simulink model "ftc_4AGENTS_sim_test"  (R2024a)
settings: Solver=VariableStepAuto  StartTime=0.0  StopTime=10  FixedStep=0.001  RelTol=1e-3
undefined symbols (not defined in the file or in its folder): param, pos_init
libraries: sim3dlib x5
settings Model: PacingRate=0.100000  Creator=antor  LastModifiedBy=antor

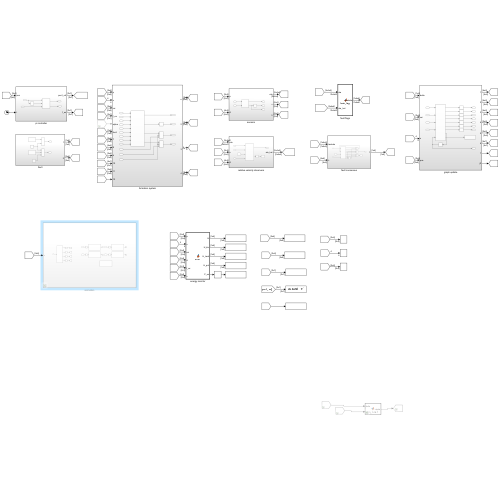
[thumbnail: Simulink's stored preview of the top-level diagram]
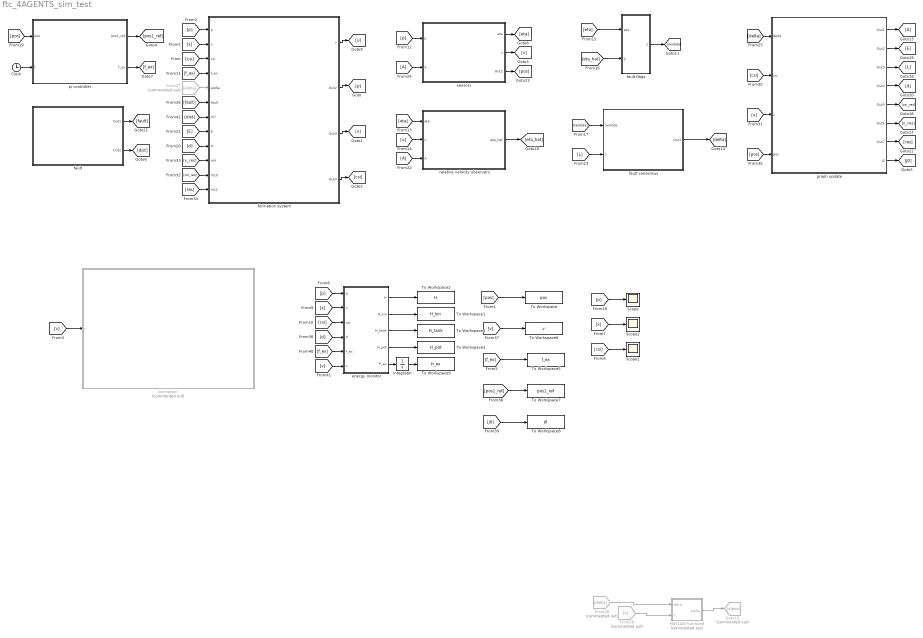
== system ftc_4AGENTS_sim_test ==
  Clock : Clock
  From22 : From
  From24 : From
  From27 : From  Commented=on  GotoTag=alpha
  From28 : From  Commented=on  GotoTag=delta
  From29 : From  Commented=on  GotoTag=x
  Goto13 : Goto
  Goto15 : Goto  Commented=on  GotoTag=alpha
  Integrator : Integrator
  MATLAB Function8 : MATLAB Function  Commented=on  TreatAsAtomicUnit=on
  Scope : Scope
  Scope1 : Scope
  Scope2 : Scope
  To Workspace : ToWorkspace  VariableName=pos  SaveFormat=Timeseries  SampleTime=param.T
  To Workspace1 : ToWorkspace  VariableName=H_kin  SaveFormat=Timeseries  SampleTime=param.T
  To Workspace2 : ToWorkspace  VariableName=H  SaveFormat=Timeseries  SampleTime=param.T
  To Workspace3 : ToWorkspace  VariableName=H_pot  SaveFormat=Timeseries  SampleTime=param.T
  To Workspace4 : ToWorkspace  VariableName=H_tank  SaveFormat=Timeseries  SampleTime=param.T
  To Workspace5 : ToWorkspace  VariableName=f_ex  SaveFormat=Timeseries  SampleTime=param.T
  To Workspace6 : ToWorkspace  VariableName=v  SaveFormat=Timeseries  SampleTime=param.T
  To Workspace7 : ToWorkspace  VariableName=pos1_ref  SaveFormat=Timeseries  SampleTime=param.T
  To Workspace8 : ToWorkspace  VariableName=j0  SaveFormat=Timeseries  SampleTime=param.T
  To Workspace9 : ToWorkspace  VariableName=H_ex  SaveFormat=Timeseries  SampleTime=param.T
  animation : Subsystem  Commented=on
  energy monitor : MATLAB Function  TreatAsAtomicUnit=on
  fault : Subsystem
  fault consensus : Subsystem
  fault flags : MATLAB Function  TreatAsAtomicUnit=on
  formation system : Subsystem
  graph update : Subsystem
  pi controller : Subsystem
  relative velocity observers : Subsystem
  sensors : Subsystem
  wires:
  energy monitor/1(H) -> To Workspace2/1
  energy monitor/2(H_kin) -> To Workspace1/1
  energy monitor/4(H_pot) -> To Workspace3/1
  energy monitor/3(H_tank) -> To Workspace4/1
  [x] -> energy monitor/2(x)
  [csi] -> energy monitor/3(csi)
  [p] -> energy monitor/1(p)
  [eta] -> fault flags/1(eta)
  [eta_hat] -> fault flags/2(eta_hat)
  fault flags/1(lambda) -> [lambda]
  MATLAB Function8/1(alpha) -> Goto15/1
  From28/1 -> MATLAB Function8/1(delta)
  From29/1 -> MATLAB Function8/2(x)
  [d] -> energy monitor/4(d)
  [lambda] -> fault consensus/1(lambda)
  [L] -> fault consensus/2(L)
  fault consensus/1(Out1) -> [delta]
  [eta] -> relative velocity observers/1(eta)
  [u] -> relative velocity observers/2(u)
  From22/1 -> relative velocity observers/3(A)
  relative velocity observers/1(eta_hat) -> [eta_hat]
  [p] -> sensors/1(p)
  From24/1 -> sensors/2(A)
  sensors/1(eta) -> [eta]
  sensors/3(Out2) -> [pos]
  [pos] -> pi controller/1(pos)
  Clock/1 -> pi controller/2(t)
  pi controller/2(f_ex) -> [f_ex]
  [p] -> formation system/1(p)
  [x] -> formation system/2(x)
  [csi] -> formation system/3(csi)
  [f_ex] -> formation system/4(f_ex)
  From27/1 -> formation system/5(alpha)
  [fault] -> formation system/6(fault)
  [E] -> formation system/8(E)
  [d] -> formation system/9(d)
  [x_res] -> formation system/10(In9)
  [csi_res] -> formation system/11(In10)
  [res] -> formation system/12(In11)
  formation system/1(u) -> [u]
  formation system/2(Out2) -> [p]
  formation system/3(Out3) -> [x]
  formation system/4(Out4) -> [csi]
  [delta] -> graph update/1(delta)
  [csi] -> graph update/2(csi)
  [x] -> graph update/3(x)
  [pos] -> graph update/4(pos)
  graph update/1(Out1) -> Goto13/1
  graph update/2(Out2) -> [E]
  graph update/3(Out3) -> [L]
  graph update/4(Out4) -> [d]
  graph update/5(Out5) -> [csi_res]
  graph update/6(Out6) -> [x_res]
  graph update/7(Out7) -> [res]
  [v] -> animation/1(v)
  [pos] -> To Workspace/1
  [f_ex] -> To Workspace5/1
  [p] -> Scope/1
  [x] -> Scope2/1
  [csi] -> Scope1/1
  sensors/2(v) -> [v]
  [v] -> To Workspace6/1
  pi controller/1(pos1_ref) -> [pos1_ref]
  [pos1_ref] -> To Workspace7/1
  graph update/8(j0) -> [j0]
  [j0] -> To Workspace8/1
  [v] -> energy monitor/6(v)
  [f_ex] -> energy monitor/5(f_ex)
  energy monitor/5(P_ex) -> Integrator/1
  Integrator/1 -> To Workspace9/1
  fault/1(Out1) -> [fault]
  fault/2(Out2) -> [dist]
  [dist] -> formation system/7(In7)

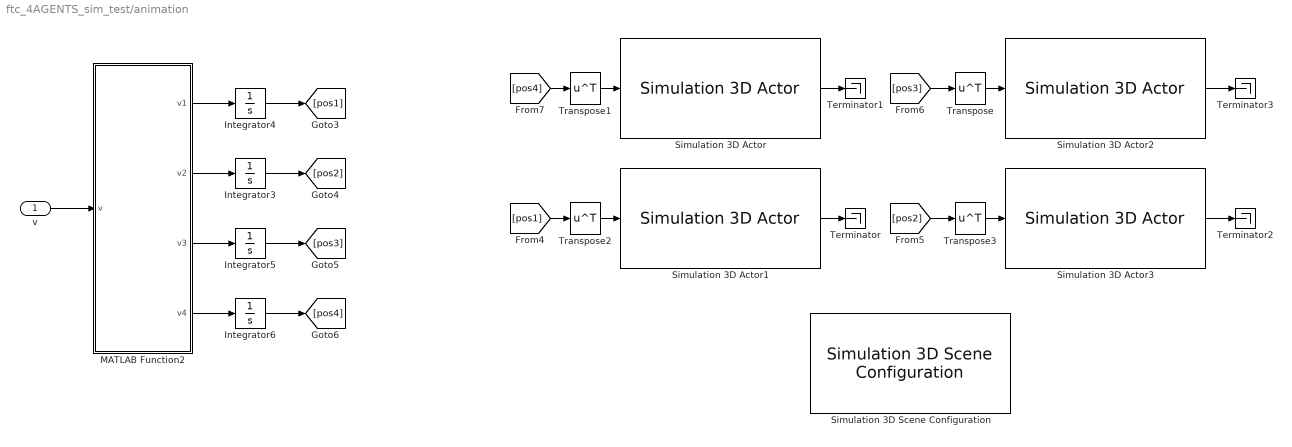
== system ftc_4AGENTS_sim_test/animation ==
  v : Inport
  Integrator3 : Integrator  InitialCondition=[pos_init(:, 2); 0]
  Integrator4 : Integrator  InitialCondition=[pos_init(:, 1); 0]
  Integrator5 : Integrator  InitialCondition=[pos_init(:, 3); 0]
  Integrator6 : Integrator  InitialCondition=[pos_init(:, 4); 0]
  MATLAB Function2 : MATLAB Function  TreatAsAtomicUnit=on
  Simulation 3D Actor : sim3dlib/Simulation 3D Actor  Priority=1  ActorName=actor4  ParentName=Scene Origin  Operation=Create at setup  InitScriptText=|  SampleTime=-1  Translation=single([0 0 0])  Rotation=single([0 0 0])  Scale=single([1 1 1])  InputsText=actor4.Translation  aMode=5  ActorTag=actor4  ActorType=Sim3dActor  ID=C
      | Actor.createShape('sphere', [1 1 1]);
      | Actor.Scale = 0.1;
      | Actor.Color = [0 0 0];
  Simulation 3D Actor1 : sim3dlib/Simulation 3D Actor  Priority=1  ActorName=actor1  ParentName=Scene Origin  Operation=Create at setup  InitScriptText=|  SampleTime=-1  Translation=single([0 0 0])  Rotation=single([0 0 0])  Scale=single([1 1 1])  InputsText=actor1.Translation  aMode=5  ActorTag=actor1  ActorType=Sim3dActor  ID=C
      | Actor.createShape('sphere', [1 1 1]);
      | Actor.Scale = 0.1;
      | Actor.Color = [0 0 1];
  Simulation 3D Actor2 : sim3dlib/Simulation 3D Actor  Priority=1  ActorName=actor3  ParentName=Scene Origin  Operation=Create at setup  InitScriptText=|  SampleTime=-1  Translation=single([0 0 0])  Rotation=single([0 0 0])  Scale=single([1 1 1])  InputsText=actor3.Translation  aMode=5  ActorTag=actor3  ActorType=Sim3dActor  ID=C
      | Actor.createShape('sphere', [1 1 1]);
      | Actor.Scale = 0.1;
      | Actor.Color = [0 0 0];
  Simulation 3D Actor3 : sim3dlib/Simulation 3D Actor  Priority=1  ActorName=actor2  ParentName=Scene Origin  Operation=Create at setup  InitScriptText=|  SampleTime=-1  Translation=single([0 0 0])  Rotation=single([0 0 0])  Scale=single([1 1 1])  InputsText=actor2.Translation  aMode=5  ActorTag=actor2  ActorType=Sim3dActor  ID=C
      | Actor.createShape('sphere', [1 1 1]);
      | Actor.Scale = 0.1;
      | Actor.Color = [0 0 0];
  Simulation 3D Scene Configuration : sim3dlib/Simulation 3D Scene Configuration  Priority=0  ProjectFormat=Default Scenes  SceneDesc=Empty scene  ProjectName=C:\Program Files\MATLAB\R2024a\toolbox\shared\sim3d_projects\automotive_project_windows\UE\WindowsNoEditor\VehicleSimulation.exe  ScenePath=/Game/Maps/HwStrght  EnableOpenDRIVE=off  vehTagList={'Custom';'Scene Origin';'actor1';'actor2';'actor3';'actor4'}  vehTag=Scene Origin  FreeCameraInitialTranslation=[2.5, 2.5, 15]  FreeCameraDefaultInitialTranslation=[-6, 0, 2]  FreeCameraInitialRotation=[90, -90, 0]  FreeCameraDefaultInitialRotation=[0, -15, 0]  OpVisEn=off  Ts=.02  EnableWindow=on  EnableRemoteAccess=off  EnableWeather=off  SunAzimuth=90  SunAltitude=40.0  EnableGeospatialSun=off  Latitude=0  Longitude=0  Date=2023-01-01  Time=10:30:00  GeoTimeZone=-5.0  SunDaylightSaving=off  wind=1  clouds=10  EnableVolumetricClouds=off  CloudCoverage=0  CloudAltitude=6  fog=0  rain=0  RaindropsEffect=off  SnowDensity=0  EnableGeospatial=off  UseTrueOrigin=off  OriginHeight=200  OriginLatitude=40.744652  OriginLongitude=-73.988864  MapStyle=Aerial  AdditionalAssetIDs=[]  UseAdvancedSunSky=off  SolarTime=11  TimeZone=-5  Day=21  Month=9  Year=2022  UseDaylightSavingTime=on  DSTStartDay=10  DSTStartMonth=3  DSTEndDay=3  DSTEndMonth=11  DSTSwitchHour=2  sensorTag=MainCamera1  sensorId=1  sensorName=MainCamera1  mountLoc=Origin  offsetFlag=off  tmountOffset=[0, 0, 0]  rmountOffset=[0, 0, 0]  HorizontalResolution=1280  VerticalResolution=720  HorizontalFOV=60  mountPoint=[0 0 0]  mountOrientation=[0 0 0]  aMode=5  ID=1  GeoTrigger=Inactive
      settings: LibrarySourceBlock=sl3dlib/Simulation 3D/Environment/Simulation 3D Scene Configuration
  Terminator{,1..3} (4 alike) : Terminator
  Transpose{,1..3} (4 alike) : Math  Operator=transpose
  wires:
  MATLAB Function2/2(v2) -> Integrator3/1
  Simulation 3D Actor/1 -> Terminator1/1
  [pos2] -> Transpose3/1
  Integrator5/1 -> [pos3]
  Integrator6/1 -> [pos4]
  [pos1] -> Transpose2/1
  Integrator4/1 -> [pos1]
  Integrator3/1 -> [pos2]
  MATLAB Function2/1(v1) -> Integrator4/1
  Simulation 3D Actor3/1 -> Terminator2/1
  MATLAB Function2/3(v3) -> Integrator5/1
  Transpose3/1 -> Simulation 3D Actor3/1
  Transpose2/1 -> Simulation 3D Actor1/1
  Transpose/1 -> Simulation 3D Actor2/1
  Transpose1/1 -> Simulation 3D Actor/1
  MATLAB Function2/4(v4) -> Integrator6/1
  Simulation 3D Actor2/1 -> Terminator3/1
  [pos4] -> Transpose1/1
  [pos3] -> Transpose/1
  Simulation 3D Actor1/1 -> Terminator/1
  v/1 -> MATLAB Function2/1(v)

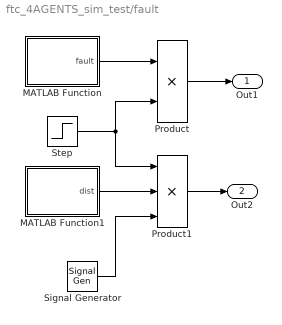
== system ftc_4AGENTS_sim_test/fault ==
  MATLAB Function : MATLAB Function  TreatAsAtomicUnit=on
  MATLAB Function1 : MATLAB Function  TreatAsAtomicUnit=on
  Product : Product
  Product1 : Product  Inputs=3
  Signal Generator : SignalGenerator  WaveForm=random  Frequency=0.2  Units=rad/sec
  Step : Step  Time=param.fault_time+100  SampleTime=0
  Out1 : Outport
  Out2 : Outport  Port=2
  wires:
  Step/1 -> Product1/1, Product/2
  MATLAB Function/1(fault) -> Product/1
  Product/1 -> Out1/1
  MATLAB Function1/1(dist) -> Product1/2
  Product1/1 -> Out2/1
  Signal Generator/1 -> Product1/3

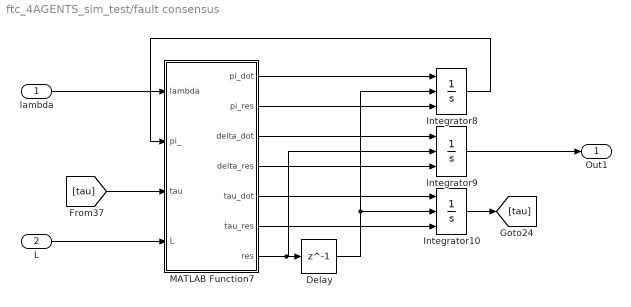
== system ftc_4AGENTS_sim_test/fault consensus ==
  lambda : Inport
  L : Inport  Port=2
  Delay : Delay  DelayLength=1
  Integrator10 : Integrator  ExternalReset=rising  InitialConditionSource=external
  Integrator8 : Integrator  ExternalReset=rising  InitialConditionSource=external
  Integrator9 : Integrator  ExternalReset=rising  InitialConditionSource=external
  MATLAB Function7 : MATLAB Function  TreatAsAtomicUnit=on
  Out1 : Outport
  wires:
  MATLAB Function7/3(delta_dot) -> Integrator9/1
  MATLAB Function7/7(res) -> Integrator9/2, Delay/1
  MATLAB Function7/1(pi_dot) -> Integrator8/1
  MATLAB Function7/6(tau_res) -> Integrator10/3
  MATLAB Function7/5(tau_dot) -> Integrator10/1
  Integrator9/1 -> Out1/1
  MATLAB Function7/2(pi_res) -> Integrator8/3
  Integrator8/1 -> MATLAB Function7/2(pi_)
  Delay/1 -> Integrator8/2, Integrator10/2
  MATLAB Function7/4(delta_res) -> Integrator9/3
  Integrator10/1 -> [tau]
  [tau] -> MATLAB Function7/3(tau)
  L/1 -> MATLAB Function7/4(L)
  lambda/1 -> MATLAB Function7/1(lambda)

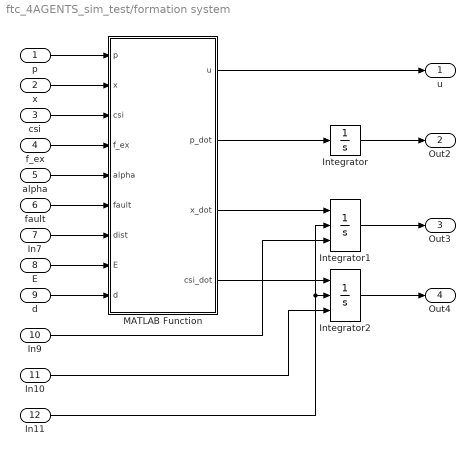
== system ftc_4AGENTS_sim_test/formation system ==
  p : Inport
  x : Inport  Port=2
  csi : Inport  Port=3
  f_ex : Inport  Port=4
  alpha : Inport  Port=5
  fault : Inport  Port=6
  In7 : Inport  Port=7
  E : Inport  Port=8
  d : Inport  Port=9
  In9 : Inport  Port=10
  In10 : Inport  Port=11
  In11 : Inport  Port=12
  Integrator : Integrator  InitialCondition=zeros(2, param.N)
  Integrator1 : Integrator  ExternalReset=rising  InitialConditionSource=external  InitialCondition=50*ones(1, param.N)
  Integrator2 : Integrator  ExternalReset=rising  InitialConditionSource=external  InitialCondition=param.csi_init
  MATLAB Function : MATLAB Function  TreatAsAtomicUnit=on
  u : Outport
  Out2 : Outport  Port=2
  Out3 : Outport  Port=3
  Out4 : Outport  Port=4
  wires:
  MATLAB Function/2(p_dot) -> Integrator/1
  MATLAB Function/4(csi_dot) -> Integrator2/1
  MATLAB Function/3(x_dot) -> Integrator1/1
  f_ex/1 -> MATLAB Function/4(f_ex)
  E/1 -> MATLAB Function/8(E)
  In11/1 -> Integrator1/2, Integrator2/2
  In9/1 -> Integrator1/3
  Integrator/1 -> Out2/1
  alpha/1 -> MATLAB Function/5(alpha)
  d/1 -> MATLAB Function/9(d)
  fault/1 -> MATLAB Function/6(fault)
  Integrator2/1 -> Out4/1
  x/1 -> MATLAB Function/2(x)
  MATLAB Function/1(u) -> u/1
  p/1 -> MATLAB Function/1(p)
  In10/1 -> Integrator2/3
  csi/1 -> MATLAB Function/3(csi)
  Integrator1/1 -> Out3/1
  In7/1 -> MATLAB Function/7(dist)

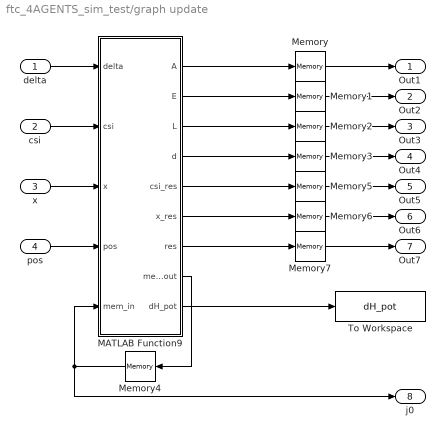
== system ftc_4AGENTS_sim_test/graph update ==
  delta : Inport
  csi : Inport  Port=2
  x : Inport  Port=3
  pos : Inport  Port=4
  MATLAB Function9 : MATLAB Function  TreatAsAtomicUnit=on
  Memory : Memory  InitialCondition=param.A
  Memory1 : Memory  InitialCondition=param.E
  Memory2 : Memory  InitialCondition=param.L
  Memory3 : Memory  InitialCondition=param.d
  Memory4 : Memory
  Memory5 : Memory  InitialCondition=param.csi_init
  Memory6 : Memory  InitialCondition=param.x_init
  Memory7 : Memory
  To Workspace : ToWorkspace  VariableName=dH_pot  SaveFormat=Timeseries  SampleTime=-1
  Out1 : Outport
  Out2 : Outport  Port=2
  Out3 : Outport  Port=3
  Out4 : Outport  Port=4
  Out5 : Outport  Port=5
  Out6 : Outport  Port=6
  Out7 : Outport  Port=7
  j0 : Outport  Port=8
  wires:
  MATLAB Function9/1(A) -> Memory/1
  Memory/1 -> Out1/1
  MATLAB Function9/3(L) -> Memory2/1
  Memory4/1 -> j0/1, MATLAB Function9/5(mem_in)
  MATLAB Function9/5(csi_res) -> Memory5/1
  MATLAB Function9/6(x_res) -> Memory6/1
  MATLAB Function9/2(E) -> Memory1/1
  MATLAB Function9/4(d) -> Memory3/1
  MATLAB Function9/8(mem_out) -> Memory4/1
  Memory1/1 -> Out2/1
  Memory3/1 -> Out4/1
  MATLAB Function9/7(res) -> Memory7/1
  Memory2/1 -> Out3/1
  x/1 -> MATLAB Function9/3(x)
  Memory6/1 -> Out6/1
  Memory5/1 -> Out5/1
  csi/1 -> MATLAB Function9/2(csi)
  Memory7/1 -> Out7/1
  delta/1 -> MATLAB Function9/1(delta)
  pos/1 -> MATLAB Function9/4(pos)
  MATLAB Function9/9(dH_pot) -> To Workspace/1

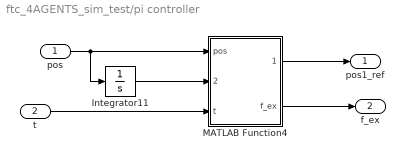
== system ftc_4AGENTS_sim_test/pi controller ==
  pos : Inport
  t : Inport  Port=2
  Integrator11 : Integrator
  MATLAB Function4 : MATLAB Function  TreatAsAtomicUnit=on
  pos1_ref : Outport
  f_ex : Outport  Port=2
  wires:
  t/1 -> MATLAB Function4/3(t)
  pos/1 -> Integrator11/1, MATLAB Function4/1(pos)
  Integrator11/1 -> MATLAB Function4/2(pos_int)
  MATLAB Function4/2(f_ex) -> f_ex/1
  MATLAB Function4/1(pos1_ref) -> pos1_ref/1

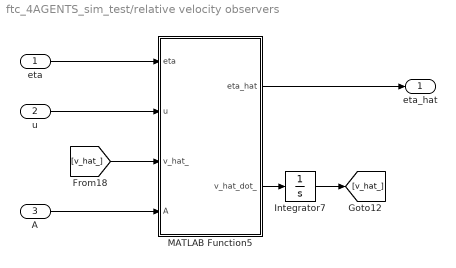
== system ftc_4AGENTS_sim_test/relative velocity observers ==
  eta : Inport
  u : Inport  Port=2
  A : Inport  Port=3
  Integrator7 : Integrator  InitialCondition=zeros(2*param.N, param.N)
  MATLAB Function5 : MATLAB Function  TreatAsAtomicUnit=on
  eta_hat : Outport
  wires:
  MATLAB Function5/1(eta_hat) -> eta_hat/1
  [v_hat_] -> MATLAB Function5/3(v_hat_)
  A/1 -> MATLAB Function5/4(A)
  eta/1 -> MATLAB Function5/1(eta)
  u/1 -> MATLAB Function5/2(u)
  Integrator7/1 -> [v_hat_]
  MATLAB Function5/2(v_hat_dot_) -> Integrator7/1

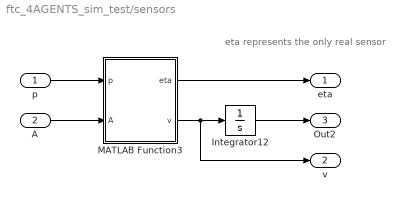
== system ftc_4AGENTS_sim_test/sensors ==
  note: eta represents the only real sensor
  p : Inport
  A : Inport  Port=2
  Integrator12 : Integrator  InitialCondition=param.pos_init
  MATLAB Function3 : MATLAB Function  TreatAsAtomicUnit=on
  eta : Outport
  v : Outport  Port=2
  Out2 : Outport  Port=3
  wires:
  MATLAB Function3/2(v) -> v/1, Integrator12/1
  MATLAB Function3/1(eta) -> eta/1
  Integrator12/1 -> Out2/1
  p/1 -> MATLAB Function3/1(p)
  A/1 -> MATLAB Function3/2(A)

== matlab function ftc_4AGENTS_sim_test/fault flags ==
  data: eta input; lambda output; eta_hat input; param parameter
function lambda = fault_flag(eta, eta_hat, param)
    N = 4;
    theta = param.theta;

    lambda = zeros(1, N, N);
    
    for i = 1:N
        for j = 1:N
            lambda(:, i, j) = norm(eta(:, i, j) - eta_hat(:, i, j)) > theta;
        end
    end

    test = lambda(:, 1, :);
end

== matlab function ftc_4AGENTS_sim_test/fault consensus/MATLAB Function7 ==
  data: lambda input; pi_ input; tau input; L input; pi_dot output; pi_res output; delta_dot output; delta_res output; tau_dot output; tau_res output; param parameter; res output
function [pi_dot, pi_res, delta_dot, delta_res, tau_dot, tau_res, res] = fault_cons(lambda, pi_, tau, L, param)
    N = 4;
    tau_star = param.tau_star;

    pi_dot = zeros(N*N, 1);
    pi_dot(:, 1) = -2*kron(L, eye(N))*pi_;
    delta_dot = zeros(1, N);
    tau_dot = 1;

    temp = squeeze(lambda).';
    pi_res = temp(:);
    delta_res = zeros(1, N);
    for i = 1:N
        [max_delta, delta_res(i)] = max(pi_(((i-1)*N + 1):i*N));
        if max_delta <= 0.1
            delta_res(i) = 0;
        end
    end
    tau_res = 0;

    res = tau >= tau_star;
end

== matlab function ftc_4AGENTS_sim_test/MATLAB Function8 ==
  data: alpha output; delta input; x input; param parameter
function alpha = en_transf(delta, x, param)
    N = 4;

    j0 = delta(1);

    alpha = zeros(N, N);
    csi_init = param.csi_init;
    if j0 > 0.9
    %     n1 = mod(j0+N-2, N)+1;
    %     n2 = mod(j0, N)+1;
    %     n3 = mod(j0+1, N)+1;
    % 
    %     for i = 1:N
    %         if x(i) >= 1
    %             alpha(i, 1:3) = 0.00001;
    %         end
    %     end
    end

    
end

== matlab function ftc_4AGENTS_sim_test/graph update/MATLAB Function9 ==
  data: delta input; csi input; x input; pos input; mem_in input; param parameter; A output; E output; L output; d output; csi_res output; x_res output; res output; mem_out output; dH_pot output
function [A, E, L, d, csi_res, x_res, res, mem_out, dH_pot] = graph_upd(delta, csi, x, pos, mem_in, param)
    N = 4;
    pos_init = param.pos_init;
    K = param.K;

    j0 = delta(1);
    if mem_in ~= 0
        j0 = mem_in;
    end

    A = zeros(N);
    A(:, :) = param.A;
    E = zeros(N);
    E(:, :) = param.E;
    L = zeros(N);
    L(:, :) = param.L;
    d = zeros(2, N);
    d(:, :) = param.d;
    csi_res = zeros(2, N);
    csi_res(:, :) = param.csi_init;
    x_res = zeros(N, 1);
    x_res(:) = param.x_init;
    res = 0;
    mem_out = 0;
    dH_pot = 0;

    if j0 > 0.9
        mem_out = j0;

        n1 = mod(j0+N-2, N)+1;
        n2 = mod(j0, N)+1;
        n3 = mod(j0+1, N)+1;

        A_new = A;
        A_new(j0, :) = zeros(1, N);
        A_new(:, j0) = zeros(N, 1);

        temp = zeros(1, N);
        temp(n2) = 1;
        A_new(n1, :) = A_new(n1, :) + temp;
        A_new(:, n1) = A_new(:, n1) + temp.';

        edges = [];
        for i = 1:N
            for j = i+1:N
                if A_new(i, j) ~= 0
                    edges = [edges; i, j];
                end
            end
        end
        E_new = zeros(N);
        for k = 1:size(edges, 1)
            E_new(edges(k, 1), k) = -1;
            E_new(edges(k, 2), k) = 1;
        end

        L_new = diag(sum(A_new, 2)) - A_new;

        pos_rest = pos_init;
        pos_rest(:, n1) = pos_init(:, n1) + (pos_init(:, j0) - pos_init(:, n1))*cos(pi/3) + (pos_init(:, n3) - pos_init(:, n1))*(1-sin(pi/3));
        d_new = zeros(2, N);
        for j = 1:N
            for i = 1:N
                d_new(:, j) = d_new(:, j) + E_new(i, j)*pos_rest(:, i);
            end
        end

        dH_pot = 0;
        for j = 1:N
            dH_pot = dH_pot - 1/2*(csi(:, j)-d(:, j)).'*K(:, :, j)*(csi(:, j)-d(:, j));
        end 
        csi_res = zeros(2, N);
        for j = 1:N
            for i = 1:N
                csi_res(:, j) = csi_res(:, j) + E_new(i, j)*pos(:, i);
            end
        end
        for j = 1:N
            dH_pot = dH_pot + 1/2*(csi_res(:, j)-d_new(:, j)).'*K(:, :, j)*(csi_res(:, j)-d_new(:, j));
        end 
        res = 1;

        H_tank = zeros(1, N);
        for i = 1:N
            H_tank(i) = 1/2*x(i)^2;
        end        
        % for i = 1:N
        %     x_res(i) = sqrt(1/2*(H_tank-dH_pot));
        % end

        x_res(j0) = x(j0);
        x_res(n1) = sqrt(H_tank(n1) + H_tank(n2) - dH_pot);
        x_res(n2) = sqrt(H_tank(n1) + H_tank(n2) - dH_pot);
        x_res(n3) = x(n3);

        E = E_new;
        A = A_new;
        L = L_new;
        d = d_new;
    end
end

== matlab function ftc_4AGENTS_sim_test/fault/MATLAB Function ==
  data: fault output; param parameter
function fault = fault(param)
N = 4;
fault_i = param.fault_i;
fault_perc = param.fault_perc;

fault = zeros(1, N);
fault(fault_i) = fault_perc/100;
end

== matlab function ftc_4AGENTS_sim_test/fault/MATLAB Function1 ==
  data: dist output; param parameter
function dist = dist(param)
N = 4;
fault_i = param.fault_i;
dist_amp = param.dist_amp;

dist = zeros(2, N);
dist(:, fault_i) = dist_amp*rand(2, 1);
end

== matlab function ftc_4AGENTS_sim_test/energy monitor ==
  data: p input; H output; x input; csi input; d input; f_ex input; v input; H_kin output; H_tank output; H_pot output; param parameter; P_ex output
function [H, H_kin, H_tank, H_pot, P_ex] = ener(p, x, csi, d, f_ex, v, param)
    N = 4;
    M = param.M;
    K = param.K;

    H_kin = zeros(1, N);
    H_tank = zeros(1, N);
    H_pot = zeros(1, N);

    for i = 1:N
        H_kin(i) = 1/2*p(:, i).'*(M(:, :, i)\p(:, i));
        H_tank(i) = 1/2*x(i)*x(i);
    end

    for j = 1:N
        H_pot(j) = 1/2*(csi(:, j)-d(:, j)).'*K(:, :, j)*(csi(:, j)-d(:, j));
    end

    H = sum([H_kin; H_pot; H_tank], 1);

    P_ex = f_ex.'*v(:, 1);
end

== matlab function ftc_4AGENTS_sim_test/formation system/MATLAB Function ==
  data: p input; u output; p_dot output; x input; csi input; f_ex input; alpha input; fault input; dist input; E input; d input; x_dot output; csi_dot output; param parameter
function [u, p_dot, x_dot, csi_dot] = sys(p, x, csi, f_ex, alpha, fault, dist, E, d, param)
    N = 4;
    K = param.K;
    M = param.M;
    B = param.B;

    r = zeros(1, 2, N);
    h = zeros(1, 2, N, N);

    for i = 1:N
        r(:, :, i) = (B(:, :, i)*(M(:, :, i)\p(:, i))).'/x(i);
        for j = 1:N
            % h(:, :, i, j) = alpha(i, j)*(K(:, :, j)*(csi(:, j)-d(:, j))*x(i)).';
        end
    end

    u = zeros(2, N);
    p_dot = zeros(2, N);
    x_dot = zeros(1, N);
    csi_dot = zeros(2, N);

    u(:, 1) = f_ex;
    for i = 1:N
        %u(:, i) = - r(:, :, i).'*x(i);
        x_dot(:, i) = r(:, :, i)*(M(:, :, i)\p(:, i));
        for j = 1:N
            u(:, i) = u(:, i) - E(i, j)*K(1, 1, j)*(norm(csi(:, j)) - 5)*csi(:, j);
            x_dot(i) = x_dot(i) - h(:, :, i, j)*K(:, :, j)*(csi(:, j) - d(:, j));
            csi_dot(:, j) = csi_dot(:, j) + E(i, j)*(M(:, :, i)\p(:, i)) + h(:, :, i, j).'*x(i);
        end
        p_dot(:, i) = (1-fault(i))*u(:, i) - M(:, :, i)\(B(:, :, i)*p(:, i)) + dist(:, i);
    end
end

== matlab function ftc_4AGENTS_sim_test/animation/MATLAB Function2 ==
  data: v1 output; v input; v2 output; v3 output; v4 output
function [v1, v2, v3, v4] = pos_anim(v)

    v1 = [v(:, 1); 0];
    v2 = [v(:, 2); 0];
    v3 = [v(:, 3); 0];
    v4 = [v(:, 4); 0];
end

== matlab function ftc_4AGENTS_sim_test/sensors/MATLAB Function3 ==
  data: p input; A input; eta output; v output; param parameter
function [eta, v] = sens(p, A, param)
    N = 4;
    M = param.M;

    eta = zeros(2, N, N);
    v = zeros(2, N);

    for i = 1:N
        v(:, i) = M(:, :, i)\p(:, i);
    end
    for j = 1:N
         eta(:, j, :) = repmat(A(j, :), 2, 1).*(v - repmat(v(:, j), 1, N));
    end

    test = eta(:, 2, :);
end

== matlab function ftc_4AGENTS_sim_test/pi controller/MATLAB Function4 ==
  data: pos1_ref output; pos input; pos_int input; t input; f_ex output
function [pos1_ref, f_ex] = pi_contr(pos, pos_int, t)
    a = 3;
    pos1_ref = [a*cos(pi/5*t); a*sin(pi/5*t)];
    pos1_int_des = [a*sin(pi/5*t); -a*cos(pi/5*t)];

    f_ex = 40*(pos1_ref - pos(1:2, 1)) + 0.8*(pos1_int_des - pos_int(1:2, 1));
end

== matlab function ftc_4AGENTS_sim_test/relative velocity observers/MATLAB Function5 ==
  data: eta input; u input; eta_hat output; v_hat_ input; A input; param parameter; v_hat_dot_ output
function [eta_hat, v_hat_dot_] = obs(eta, u, v_hat_, A, param)
    % v_hat(:, 1, 2) is what agent 1 thinks agent 2's velocity is
    
    N = 4;
    M = param.M;
    B = param.B;
    R = param.R;

    eta_hat = zeros(2, N, N);
    v_hat_dot = zeros(2, N, N);

    v_hat = reshape(v_hat_, 2, N, []);

    for i = 1:N
        for j = 1:N
            v_hat_dot(:, i, j) = A(i, j)*(M(:, :, j)\(u(:, j) - (B(:, :, j)*v_hat(:, i, j))) + R/2*(eta(:, i, j) - v_hat(:, i, j) + v_hat(:, j, i)));
        end
    end

    for i = 1:N
        for j = 1:N
             eta_hat(:, i, j) = v_hat(:, i, j) - v_hat(:, j, i);
        end
    end

    v_hat_dot_ = reshape(v_hat_dot, [], N);
end
